simulink model "observer_controller"  (R2024a)
settings: Solver=VariableStepAuto  StartTime=0.0  StopTime=30  RelTol=1e-3
values from neighbouring files (symbols this model uses):
  A = [-1.7, -0.25, 0 ... (first row only)    [main.m]
  B = [7, 0 ... (first row only)    [main.m]
  C = [0, 1, 0 ... (first row only)    [main.m]
  K = real(R \ B' * P)    [LQR_own.m]    (also in decoupling.m = Bstar\C_star; main.m = real(inv(R)*B_bar'*P); pole_placement.m = Kbar*T)
  L = place(A',C',desired_poles)'    [main.m]
  x0 = [1 100 200]'    [main.m]
settings Model: Creator=wyton  LastModifiedBy=chint
settings SolverCC: AlgebraicLoopSolver=TrustRegion
settings DebuggingCC: UnconnectedInputMsg=warning  UnconnectedOutputMsg=warning  UnconnectedLineMsg=warning
settings ModelReferenceCC: EnableRefExpFcnMdlSchedulingChecks=on
settings RTWCC: GPUComputeCapability=3.5

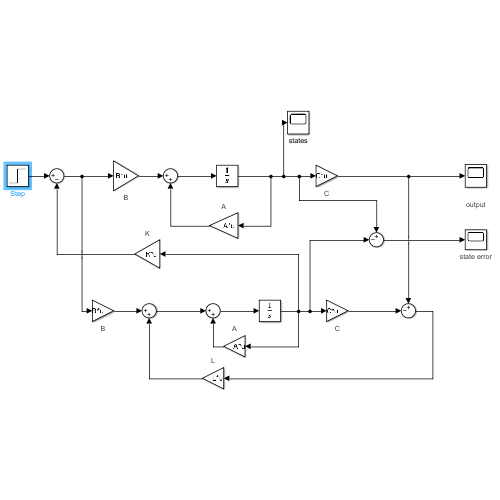
[thumbnail: Simulink's stored preview of the top-level diagram]
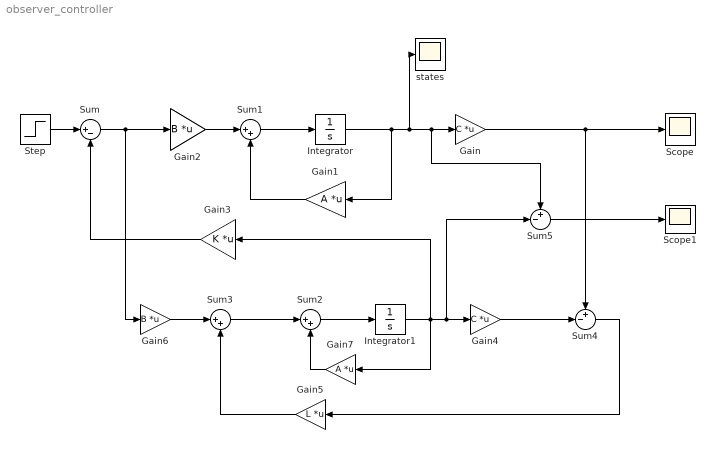
== system observer_controller ==
  Gain : Gain  Gain=C  Multiplication=Matrix(K*u)
      settings: AttributesFormatString=C
  Gain1 : Gain  Gain=A  Multiplication=Matrix(K*u)
      settings: AttributesFormatString=A
  Gain2 : Gain  Tag=B  Gain=B  Multiplication=Matrix(K*u)
      settings: AttributesFormatString=B
  Gain3 : Gain  Gain=K  Multiplication=Matrix(K*u)
      settings: AttributesFormatString=K
  Gain4 : Gain  Gain=C  Multiplication=Matrix(K*u)
      settings: AttributesFormatString=C
  Gain5 : Gain  Gain=L  Multiplication=Matrix(K*u)
      settings: AttributesFormatString=L
  Gain6 : Gain  Gain=B  Multiplication=Matrix(K*u)
      settings: AttributesFormatString=B
  Gain7 : Gain  Gain=A  Multiplication=Matrix(K*u)
      settings: AttributesFormatString=A
  Integrator : Integrator  InitialCondition=x0
  Integrator1 : Integrator
  Scope : Scope
      settings: AttributesFormatString=output
  Scope1 : Scope
      settings: AttributesFormatString=state error
  Step : Step  Time=0  Before=[0,0]  After=[0;1]  SampleTime=0
  Sum : Sum  Inputs=|+-
  Sum1 : Sum  Inputs=|++
  Sum2 : Sum  Inputs=|++
  Sum3 : Sum  Inputs=|++
  Sum4 : Sum  Inputs=+-|
  Sum5 : Sum  Inputs=+-|
  states : Scope
  wires:
  Step/1 -> Sum/1
  Sum/1 -> Gain6/1, Gain2/1
  Sum1/1 -> Integrator/1
  Gain2/1 -> Sum1/1
  Integrator/1 -> Gain1/1, states/1, Sum5/1, Gain/1
  Gain1/1 -> Sum1/2
  Gain/1 -> Sum4/1, Scope/1
  Gain3/1 -> Sum/2
  Gain6/1 -> Sum3/1
  Gain5/1 -> Sum3/2
  Sum3/1 -> Sum2/1
  Gain7/1 -> Sum2/2
  Sum2/1 -> Integrator1/1
  Integrator1/1 -> Gain3/1, Sum5/2, Gain4/1, Gain7/1
  Gain4/1 -> Sum4/2
  Sum5/1 -> Scope1/1
  Sum4/1 -> Gain5/1
